simulink model "smc_dtsmc"  (R2022a)
settings: Solver=VariableStepAuto  StartTime=0.0  StopTime=50  RelTol=1e-3
values from neighbouring files (symbols this model uses):
  A = sysd.A    [init.m]
  alpha = 0.002    [init.m]
  B = sysd.B    [init.m]
  beta = 0.001    [init.m]
  c1 = [0.25 ... (first row only)    [init.m]
  c2 = 10*[ 0.25 ... (first row only)    [init.m]
  d = 1.0    (= 1)    [init.m]
  d1 = 0.5*c1'*B*(dmax + dmin)    [init.m]
  d2 = 0.5*c2'*A*B*(dmax + dmin)    [init.m]
  del_d1 = 0.5*abs(c1'*B)*(dmax - dmin)    [init.m]
  del_d2 = 0.5*abs(c2'*A*B)*(dmax - dmin)    [init.m]
  epsi = 0.1    [init.m]
  ks = 0.02    [init.m]
  kv = 0.05    [init.m]
  M = 5    [init.m]
  s0 = 1.0    (= 1)    [init.m]
  Ts = 5E-3    (= 0.005)    [init.m]
settings Model: Creator=Admin  LastModifiedBy=Admin

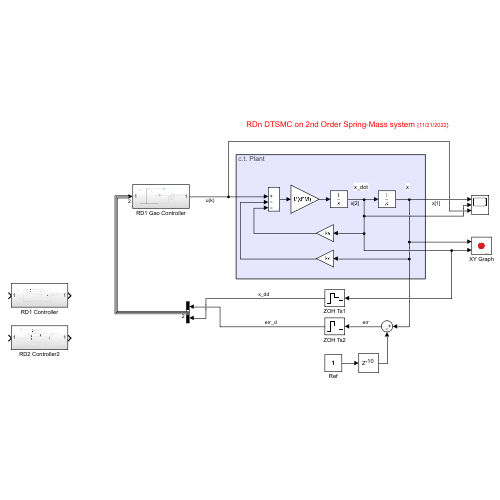
[thumbnail: Simulink's stored preview of the top-level diagram]
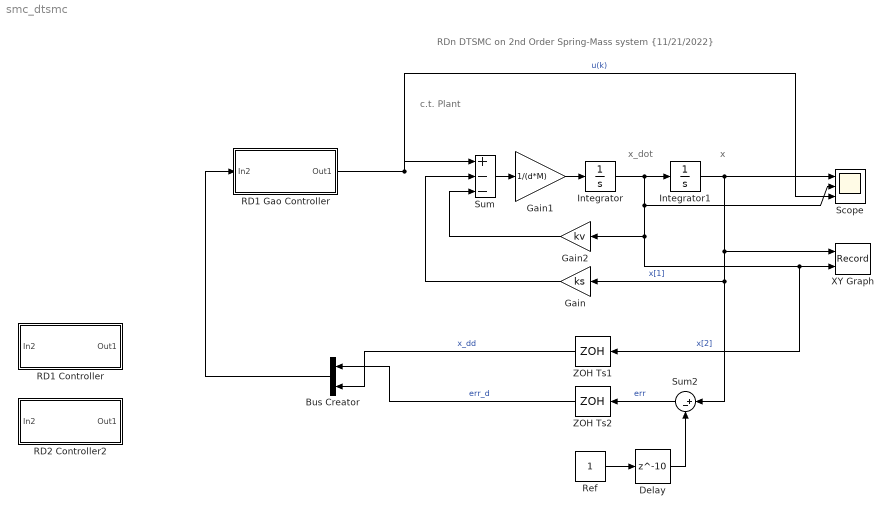
== system smc_dtsmc ==
  note: RDn DTSMC on 2nd Order Spring-Mass system {11/21/2022}
  note: c.t. Plant
  note: x
  note: x_dot
  Bus Creator : BusCreator  Inputs=2
  Delay : Delay  DelayLength=10  InitialCondition=0  SampleTime=Ts
  Gain : Gain  Gain=ks
  Gain1 : Gain  Gain=1/(d*M)
  Gain2 : Gain  Gain=kv
  Integrator : Integrator
  Integrator1 : Integrator
  RD1 Controller : Subsystem
  RD1 Gao Controller : Subsystem
  RD2 Controller2 : Subsystem
  Ref : Constant
  Scope : Scope  NumInputPorts=3
  Sum : Sum  Inputs=|+--
  Sum2 : Sum  Inputs=|+-
  XY Graph : Record  FileSettingsInternal="{\"entries\":[{\"content\":{\"excelSettings\":{\"content\":{},\"type\":\"Streamout.ExcelSettings\"}},\"type\":\"Streamout.FileSettingStorage\",\"uuid\":\"5b4049c3-9d8a-4c72-bebd-7f175cb8ba45\"}],\"packageUris\":[\"http://schema.mathworks.com/mf0/streamout_blocks/R2020a\"],\"version\":\"1.0\"}"  Layout=[1 1]  SignalsInternal="{\"entries\":[{\"content\":{\"signals\":[{\"content\":{\"blockPath\":[\"smc_dtsmc/XY Graph\"],\"channel\":[],\"dimensions\":[1],\"domain\":\"smc_dtsmc/XY Graph\",\"lineColor\":\"#a2142f\",\"plots\":[1],\"port\":1,\"sid\":[\"\"],\"signalID\":8401,\"signalName\":\"x[1]\"},\"type\":\"RecordBlkView.Signal\",\"uuid\":\"730d20da-5d88-4194-bfce-ea29c17dcd81\"},{\"content\":{\"blockPath\":[\"smc_dtsmc/XY Graph\"],\"channel\":[],\"dimensions\":[1],\"domain\":\"smc_dtsmc/XY Graph\",\"lineColor\":\"#139fff\",\"plots\":[1],\"port\":2,\"sid\":[\"\"],\"signalID\":8405,\"signalName\":\"x[2]\"},\"type\":\"RecordBlkView.Signal\",\"uuid\":\"7bf86e24-aa07-438d-8d49-052770da3d9d\"}]},\"type\":\"RecordBlkView.InputSignals\",\"uuid\":\"7bb2c2a4-a656-46c0-95a0-ddecc13524d8\"}],\"packageUris\":[\"http://schema.mathworks.com/mf0/streamout_blocks/R2020a\"],\"version\":\"1.0\"}"  VisualizationBindings="{\"xyplotplugin\":{\"info\":[{\"series\":[{\"bindingParametersList\":[{\"parameter\":\"X-Axis\",\"signalID\":8401,\"signalName\":\"x[1]\"},{\"parameter\":\"Y-Axis\",\"signalID\":8405,\"signalName\":\"x[2]\"}],\"seriesID\":49075}],\"subplotID\":1}]}}"  CompatibilityTag=XY
  ZOH Ts1 : ZeroOrderHold  SampleTime=Ts
  ZOH Ts2 : ZeroOrderHold  SampleTime=Ts
  wires:
  Integrator/1 -> Scope/2, ZOH Ts1/1, XY Graph/2, Gain2/1, Integrator1/1  "x[2]"
  Gain/1 -> Sum/2
  Integrator1/1 -> Scope/1, XY Graph/1, Sum2/1, Gain/1  "x[1]"
  Sum/1 -> Gain1/1
  Gain1/1 -> Integrator/1
  Gain2/1 -> Sum/3
  RD1 Gao Controller/1(Out1) -> Scope/3, Sum/1  "u(k)"
  Sum2/1 -> ZOH Ts2/1  "err"
  Delay/1 -> Sum2/2
  Ref/1 -> Delay/1
  ZOH Ts2/1 -> Bus Creator/1  "err_d"
  ZOH Ts1/1 -> Bus Creator/2  "x_dd"
  Bus Creator/1 -> RD1 Gao Controller/1(In2)

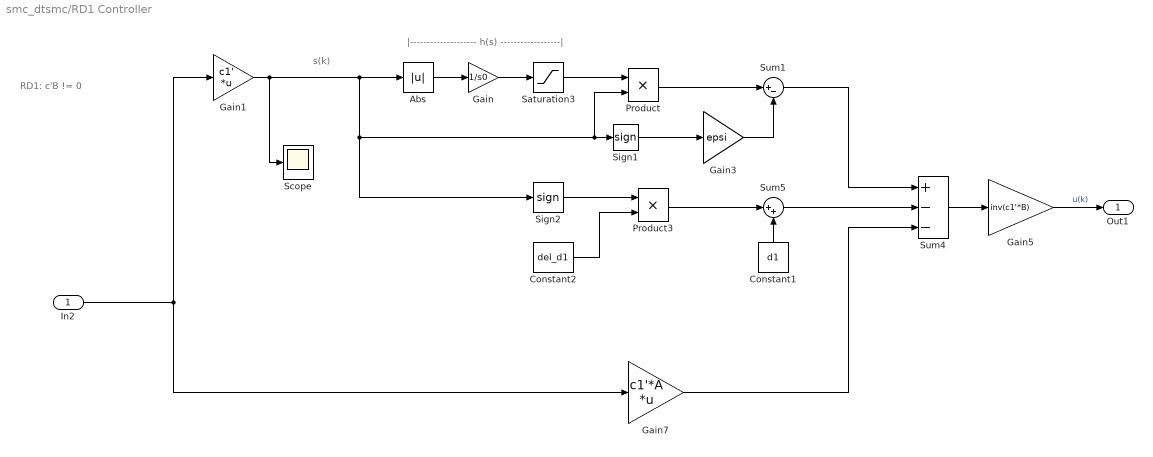
== system smc_dtsmc/RD1 Controller ==
  note: s(k)
  note: |-------------------- h(s) ------------------|
  note: RD1:
      | c'B != 0
  In2 : Inport  PortDimensions=2
  Abs : Abs  SaturateOnIntegerOverflow=off
  Constant1 : Constant  Value=d1
  Constant2 : Constant  Value=del_d1
  Gain : Gain  Gain=1/s0
  Gain1 : Gain  Gain=c1'  Multiplication=Matrix(K*u)
  Gain3 : Gain  Gain=epsi
  Gain5 : Gain  Gain=inv(c1'*B)
  Gain7 : Gain  Gain=c1'*A  Multiplication=Matrix(K*u)
  Product : Product
  Product3 : Product
  Saturation3 : Saturate  UpperLimit=1  LowerLimit=-1
  Scope : Scope
  Sign1 : Signum
  Sign2 : Signum
  Sum1 : Sum  Inputs=|+-
  Sum4 : Sum  Inputs=+--
  Sum5 : Sum  Inputs=|++
  Out1 : Outport
  wires:
  Sum4/1 -> Gain5/1
  Saturation3/1 -> Product/1
  Constant2/1 -> Product3/2
  Gain1/1 -> Abs/1, Sign2/1, Product/2, Sign1/1, Scope/1
  Product3/1 -> Sum5/1
  Sign2/1 -> Product3/1
  In2/1 -> Gain7/1, Gain1/1
  Gain/1 -> Saturation3/1
  Abs/1 -> Gain/1
  Gain5/1 -> Out1/1  "u(k)"
  Gain7/1 -> Sum4/3
  Constant1/1 -> Sum5/2
  Sum1/1 -> Sum4/1
  Product/1 -> Sum1/1
  Gain3/1 -> Sum1/2
  Sign1/1 -> Gain3/1
  Sum5/1 -> Sum4/2

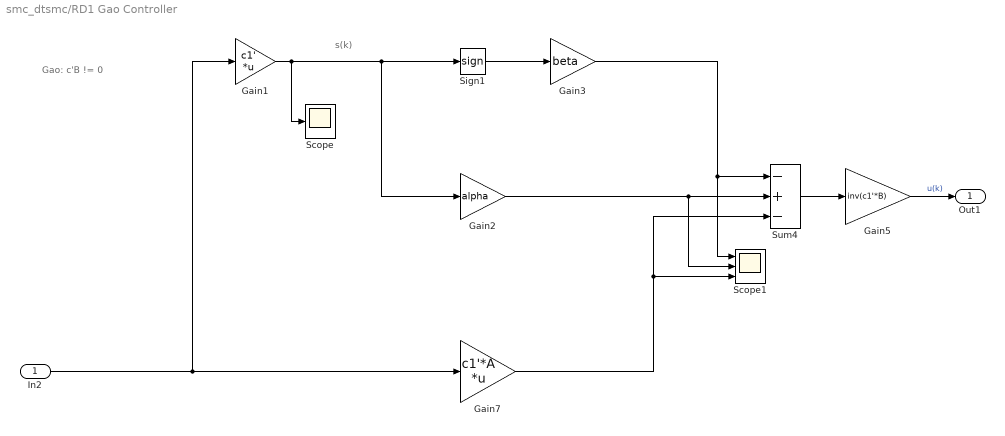
== system smc_dtsmc/RD1 Gao Controller ==
  note: s(k)
  note: Gao:
      | c'B != 0
  In2 : Inport  PortDimensions=2
  Gain1 : Gain  Gain=c1'  Multiplication=Matrix(K*u)
  Gain2 : Gain  Gain=alpha
  Gain3 : Gain  Gain=beta
  Gain5 : Gain  Gain=inv(c1'*B)
  Gain7 : Gain  Gain=c1'*A  Multiplication=Matrix(K*u)
  Scope : Scope
  Scope1 : Scope  NumInputPorts=3
  Sign1 : Signum
  Sum4 : Sum  Inputs=-+-
  Out1 : Outport
  wires:
  Sum4/1 -> Gain5/1
  Gain1/1 -> Sign1/1, Gain2/1, Scope/1
  Gain5/1 -> Out1/1  "u(k)"
  Sign1/1 -> Gain3/1
  Gain2/1 -> Scope1/2, Sum4/2
  Gain7/1 -> Scope1/3, Sum4/3
  Gain3/1 -> Scope1/1, Sum4/1
  In2/1 -> Gain1/1, Gain7/1

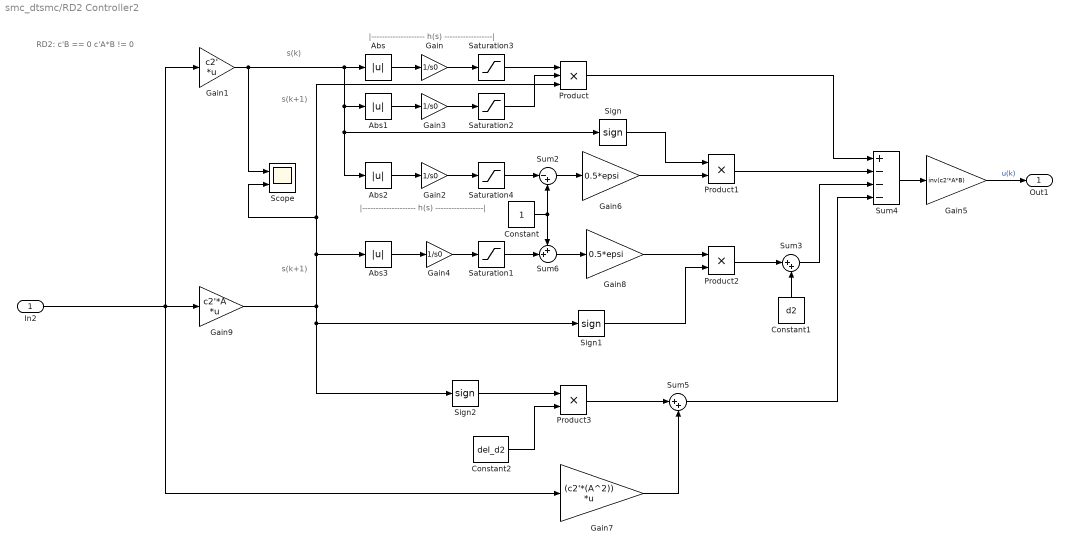
== system smc_dtsmc/RD2 Controller2 ==
  note: RD2:
      | c'B == 0
      | c'A*B != 0
  note: s(k)
  note: s(k+1)
  note: |-------------------- h(s) ------------------|
  note: |-------------------- h(s) ------------------|
  note: s(k+1)
  In2 : Inport  PortDimensions=2
  Abs{,1..3} (4 alike) : Abs  SaturateOnIntegerOverflow=off
  Constant : Constant
  Constant1 : Constant  Value=d2
  Constant2 : Constant  Value=del_d2
  Gain{,2..4} (4 alike) : Gain  Gain=1/s0
  Gain1 : Gain  Gain=c2'  Multiplication=Matrix(K*u)
  Gain5 : Gain  Gain=inv(c2'*A*B)
  Gain6 : Gain  Gain=0.5*epsi
  Gain7 : Gain  Gain=(c2'*(A^2))  Multiplication=Matrix(K*u)
  Gain8 : Gain  Gain=0.5*epsi
  Gain9 : Gain  Gain=c2'*A  Multiplication=Matrix(K*u)
  Product : Product  Inputs=3
  Product1 : Product
  Product2 : Product
  Product3 : Product
  Saturation{1..4} (4 alike) : Saturate  UpperLimit=1  LowerLimit=-1
  Scope : Scope  NumInputPorts=2
  Sign : Signum
  Sign1 : Signum
  Sign2 : Signum
  Sum2 : Sum  Inputs=|-+
  Sum3 : Sum  Inputs=|++
  Sum4 : Sum  Inputs=+---
  Sum5 : Sum  Inputs=|++
  Sum6 : Sum  Inputs=++|
  Out1 : Outport
  wires:
  Sum4/1 -> Gain5/1
  Sum2/1 -> Gain6/1
  Constant/1 -> Sum6/1, Sum2/2
  Saturation3/1 -> Product/1
  Constant2/1 -> Product3/2
  Sum5/1 -> Sum4/4
  Sign/1 -> Product1/1
  Product1/1 -> Sum4/2
  Product/1 -> Sum4/1
  Product2/1 -> Sum3/1
  Sign1/1 -> Product2/2
  Saturation2/1 -> Product/2
  Sum3/1 -> Sum4/3
  Product3/1 -> Sum5/1
  Sign2/1 -> Product3/1
  Gain6/1 -> Product1/2
  Constant1/1 -> Sum3/2
  Gain8/1 -> Product2/1
  Sum6/1 -> Gain8/1
  Saturation4/1 -> Sum2/1
  In2/1 -> Gain1/1, Gain9/1, Gain7/1
  Gain7/1 -> Sum5/2
  Gain/1 -> Saturation3/1
  Abs/1 -> Gain/1
  Abs1/1 -> Gain3/1
  Gain3/1 -> Saturation2/1
  Gain2/1 -> Saturation4/1
  Abs2/1 -> Gain2/1
  Gain5/1 -> Out1/1  "u(k)"
  Abs3/1 -> Gain4/1
  Gain4/1 -> Saturation1/1
  Saturation1/1 -> Sum6/2
  Gain9/1 -> Sign2/1, Sign1/1, Scope/2, Product/3, Abs3/1
  Gain1/1 -> Abs/1, Abs1/1, Sign/1, Abs2/1, Scope/1
